simulink model "capacity_fade_based_on_T_V_t"  (R2017a)
settings: Solver=VariableStepAuto  StartTime=0.0  StopTime=10.0  RelTol=1e-3
settings Model: Creator=srajuvel  LastModifiedBy=srajuvel

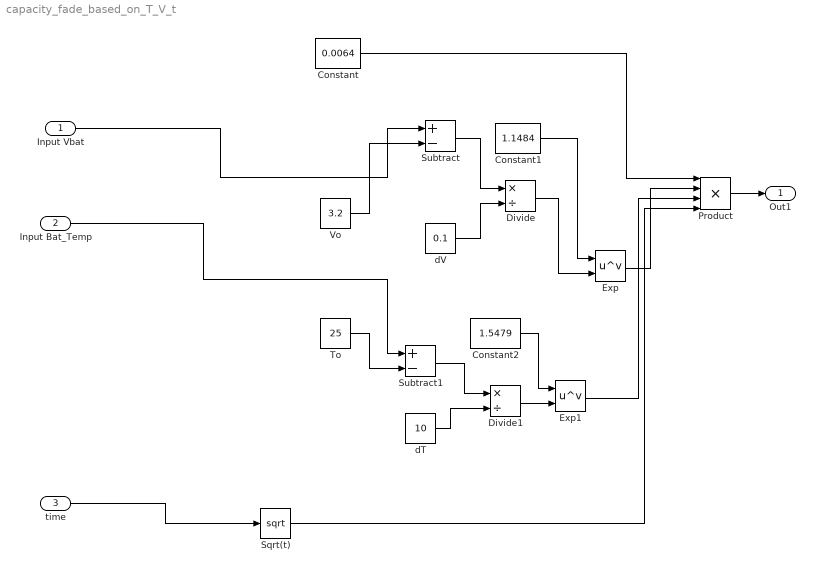
== system capacity_fade_based_on_T_V_t ==
  Input Vbat : Inport
  Input Bat_Temp : Inport  Port=2
  time : Inport  Port=3
  Constant : Constant  Value=0.0064
  Constant1 : Constant  Value=1.1484
  Constant2 : Constant  Value=1.5479
  Divide : Product  Inputs=*/
  Divide1 : Product  Inputs=*/
  Exp : Math  Operator=pow  SaturateOnIntegerOverflow=on
  Exp1 : Math  Operator=pow  SaturateOnIntegerOverflow=on
  Product : Product  Inputs=4
  Sqrt(t) : Sqrt  SaturateOnIntegerOverflow=on
  Subtract : Sum  Inputs=+-
  Subtract1 : Sum  Inputs=+-
  To : Constant  Value=25
  Vo : Constant  Value=3.2
  dT : Constant  Value=10
  dV : Constant  Value=0.1
  Out1 : Outport
  wires:
  Input Vbat/1 -> Subtract/1
  Input Bat_Temp/1 -> Subtract1/1
  Vo/1 -> Subtract/2
  Subtract/1 -> Divide/1
  dV/1 -> Divide/2
  Constant1/1 -> Exp/1
  Divide/1 -> Exp/2
  To/1 -> Subtract1/2
  Subtract1/1 -> Divide1/1
  dT/1 -> Divide1/2
  Constant2/1 -> Exp1/1
  Divide1/1 -> Exp1/2
  time/1 -> Sqrt(t)/1
  Constant/1 -> Product/1
  Exp/1 -> Product/2
  Exp1/1 -> Product/3
  Sqrt(t)/1 -> Product/4
  Product/1 -> Out1/1
